simulink model "c"  (R2012b)
settings: Solver=ode45  StartTime=0.0  StopTime=10.0  RelTol=1e-3
values from neighbouring files (symbols this model uses):
  A = [-0.4 -0.2 -0.1 -0.05 -0.01 0 0.6 1.5 3.2 4 4.1]    [labc.mat]
  V = [-5 -4 -3 -2 -1 0 1 2 3 4 5]    [labc.mat]
settings Model: Creator=ZhouHaoyu  LastModifiedBy=ZhouHaoyu

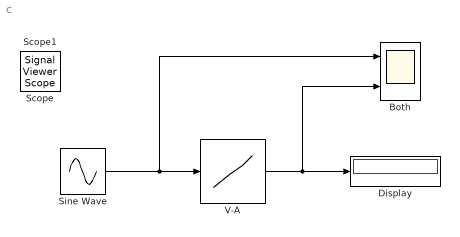
== system c ==
  Both : Scope  NumInputPorts=2
      settings: YMin=-5~-5  YMax=5~5
  Display : Display
  Sine Wave : Sin  Amplitude=5  SampleTime=0
  V-A : Lookup_n-D  NumberOfTableDimensions=1  BreakpointsForDimension1=V  Table=A  RndMeth=Simplest  InputSameDT=on
  Scope : SignalViewerScope  IOType=viewer  RefreshTime=0.035000
  Scope1 : SignalViewerScope  IOType=viewer  RefreshTime=0.035000
  wires:
  Sine Wave/1 -> Both/1, V-A/1
  V-A/1 -> Both/2, Display/1
